simulink model "EV_drive_cycle"  (R2024b)
settings: Solver=VariableStepAuto  StartTime=0.0  StopTime=765  RelTol=1e-3
settings Model: Creator=Shashwat Sinha  LastModifiedBy=Shashwat Sinha

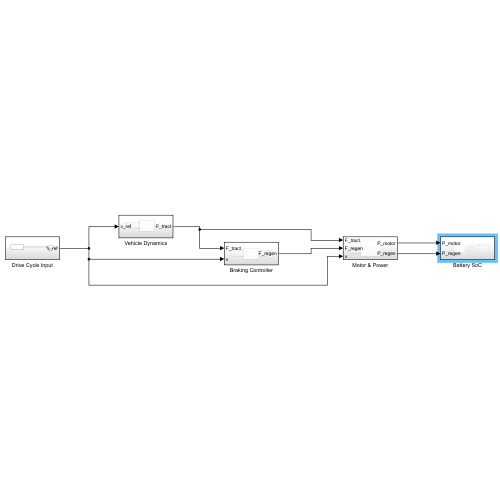
[thumbnail: Simulink's stored preview of the top-level diagram]
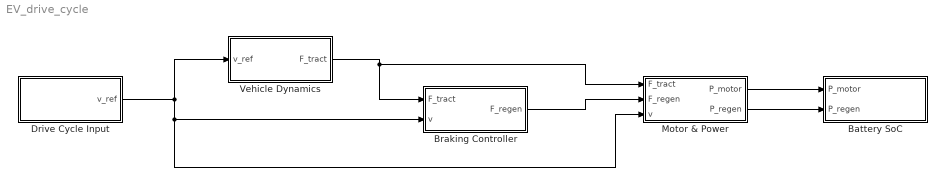
== system EV_drive_cycle ==
  Battery SoC : Subsystem
  Braking Controller : Subsystem
  Drive Cycle Input : Subsystem
  Motor & Power : Subsystem
  Vehicle Dynamics : Subsystem
  wires:
  Drive Cycle Input/1(v_ref) -> Motor & Power/3(v), Braking Controller/2(v), Vehicle Dynamics/1(v_ref)
  Vehicle Dynamics/1(F_tract) -> Motor & Power/1(F_tract), Braking Controller/1(F_tract)
  Braking Controller/1(F_regen) -> Motor & Power/2(F_regen)
  Motor & Power/1(P_motor) -> Battery SoC/1(P_motor)
  Motor & Power/2(P_regen) -> Battery SoC/2(P_regen)

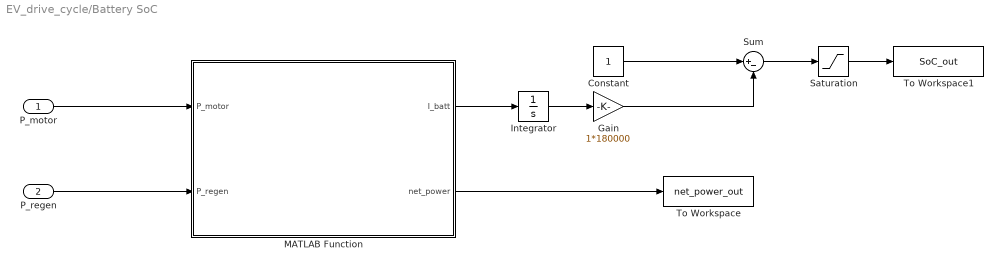
== system EV_drive_cycle/Battery SoC ==
  P_motor : Inport
  P_regen : Inport  Port=2
  Constant : Constant
  Gain : Gain  Gain=1*180000
  Integrator : Integrator
  MATLAB Function : MATLAB Function  TreatAsAtomicUnit=on
  Saturation : Saturate  UpperLimit=1  LowerLimit=0
  Sum : Sum  Inputs=|+-
  To Workspace : ToWorkspace  VariableName=net_power_out  SaveFormat=Timeseries  SampleTime=-1
  To Workspace1 : ToWorkspace  VariableName=SoC_out  SaveFormat=Timeseries  SampleTime=-1
  wires:
  MATLAB Function/1(I_batt) -> Integrator/1
  P_motor/1 -> MATLAB Function/1(P_motor)
  P_regen/1 -> MATLAB Function/2(P_regen)
  Integrator/1 -> Gain/1
  Gain/1 -> Sum/2
  Constant/1 -> Sum/1
  Sum/1 -> Saturation/1
  Saturation/1 -> To Workspace1/1
  MATLAB Function/2(net_power) -> To Workspace/1

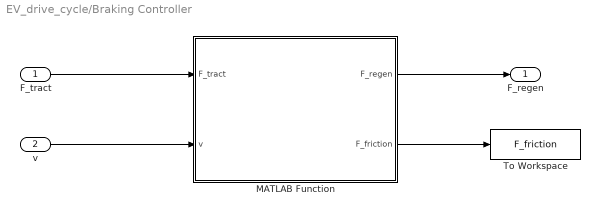
== system EV_drive_cycle/Braking Controller ==
  F_tract : Inport
  v : Inport  Port=2
  MATLAB Function : MATLAB Function  TreatAsAtomicUnit=on
  To Workspace : ToWorkspace  VariableName=F_friction  SaveFormat=Timeseries  SampleTime=-1
  F_regen : Outport
  wires:
  F_tract/1 -> MATLAB Function/1(F_tract)
  v/1 -> MATLAB Function/2(v)
  MATLAB Function/2(F_friction) -> To Workspace/1
  MATLAB Function/1(F_regen) -> F_regen/1

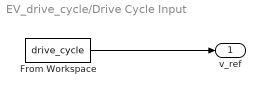
== system EV_drive_cycle/Drive Cycle Input ==
  From Workspace : FromWorkspace  VariableName=drive_cycle  SampleTime=0.1
  v_ref : Outport
  wires:
  From Workspace/1 -> v_ref/1

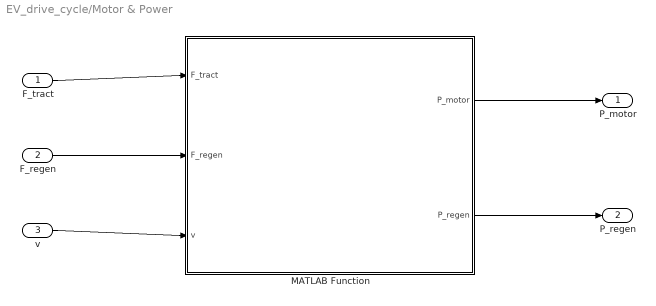
== system EV_drive_cycle/Motor & Power ==
  F_tract : Inport
  F_regen : Inport  Port=2
  v : Inport  Port=3
  MATLAB Function : MATLAB Function  TreatAsAtomicUnit=on
  P_motor : Outport
  P_regen : Outport  Port=2
  wires:
  F_tract/1 -> MATLAB Function/1(F_tract)
  F_regen/1 -> MATLAB Function/2(F_regen)
  v/1 -> MATLAB Function/3(v)
  MATLAB Function/1(P_motor) -> P_motor/1
  MATLAB Function/2(P_regen) -> P_regen/1

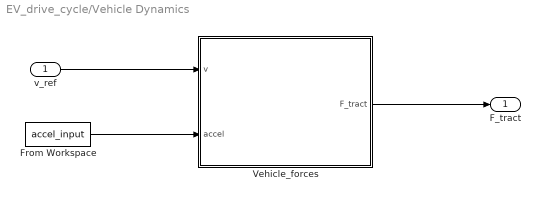
== system EV_drive_cycle/Vehicle Dynamics ==
  v_ref : Inport
  From Workspace : FromWorkspace  VariableName=accel_input  SampleTime=0.1
  Vehicle_forces : MATLAB Function  TreatAsAtomicUnit=on
  F_tract : Outport
  wires:
  From Workspace/1 -> Vehicle_forces/2(accel)
  v_ref/1 -> Vehicle_forces/1(v)
  Vehicle_forces/1(F_tract) -> F_tract/1

== matlab function EV_drive_cycle/Braking Controller/MATLAB Function ==
  data: F_tract input; F_regen output; v input; F_friction output
function [F_regen, F_friction] = braking_controller(F_tract, v)
    if F_tract >= 0
        % Accelerating — no braking
        F_regen = 0;
        F_friction = 0;
    elseif v > 15
        % Full regen
        F_regen = F_tract;
        F_friction = 0;
    elseif v > 5
        % Partial regen (linear blend)
        regen_ratio = (v - 5) / 10;
        F_regen = F_tract * regen_ratio;
        F_friction = F_tract * (1 - regen_ratio);
    else
        % Low speed — friction only
        F_regen = 0;
        F_friction = F_tract;
    end
end

== matlab function EV_drive_cycle/Vehicle Dynamics/Vehicle_forces ==
  data: v input; F_tract output; accel input
function F_tract = vehicle_dynamics(v, accel)
    % Vehicle parameters
    m = 1500;       % kg
    Cd = 0.28;
    A = 2.2;        % m^2
    rho = 1.225;    % kg/m^3
    Crr = 0.01;
    g = 9.81;

    F_aero = 0.5 * rho * Cd * A * v^2;
    F_roll = m * g * Crr;
    F_inertia = m * accel;

    F_tract = F_inertia + F_aero + F_roll;
end

== matlab function EV_drive_cycle/Motor & Power/MATLAB Function ==
  data: F_tract input; P_motor output; F_regen input; v input; P_regen output
function [P_motor, P_regen] = motor_power(F_tract, F_regen, v)
    eta_motor = 0.92;    % motoring efficiency
    eta_regen = 0.85;    % regen efficiency (slightly lower)

    if F_tract >= 0
        P_motor = (F_tract * v) / eta_motor;  % power drawn from battery
        P_regen = 0;
    else
        P_motor = 0;
        P_regen = abs(F_regen) * v * eta_regen;  % power returned to battery
    end
end

== matlab function EV_drive_cycle/Battery SoC/MATLAB Function ==
  data: P_motor input; I_batt output; P_regen input; net_power output
function [I_batt, net_power] = battery_current(P_motor, P_regen)
    V_nominal = 360;   % Volts (typical EV pack)

    net_power = P_motor - P_regen;  % positive = discharging, negative = charging
    I_batt = net_power / V_nominal; % Amperes
end
